simulink model "ss_vec2angles_test"  (R2018b)
settings: Solver=VariableStepAuto  StartTime=0.0  StopTime=10.0  RelTol=1e-3
libraries: vrlib x2, ss_angles_2_vec x1, two_norm x1, ss_vec_2_angles x1
settings Model: Creator=Taylor  LastModifiedBy=Taylor

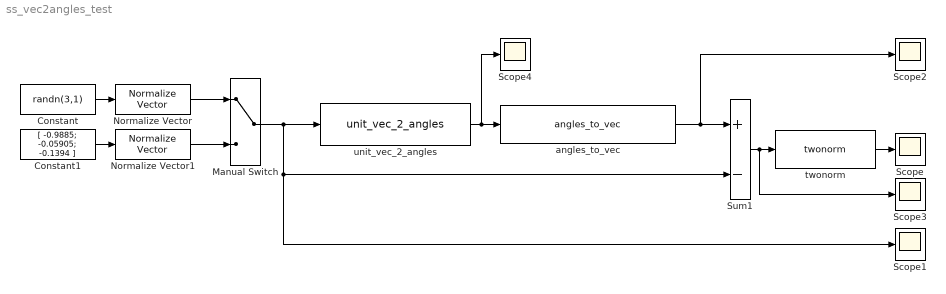
== system ss_vec2angles_test ==
  Constant : Constant  Value=randn(3,1)
  Constant1 : Constant  Value=[ -0.9885; -0.05905; -0.1394 ]
  Manual Switch : ManualSwitch
  Normalize Vector : vrlib/Utilities/Normalize Vector  maxzero=0
      settings: SourceProductName=Simulink 3D Animation  SourceProductBaseCode=VR
  Normalize Vector1 : vrlib/Utilities/Normalize Vector  maxzero=0
      settings: SourceProductName=Simulink 3D Animation  SourceProductBaseCode=VR
  Scope{,1..4} (5 alike) : Scope
  Sum1 : Sum  Inputs=+-
  angles_to_vec : ss_angles_2_vec/angles_to_vec  SystemSampleTime=-1
  twonorm : two_norm/twonorm  SystemSampleTime=-1
  unit_vec_2_angles : ss_vec_2_angles/unit_vec_2_angles  SystemSampleTime=-1
  wires:
  unit_vec_2_angles/1 -> Scope4/1, angles_to_vec/1
  Sum1/1 -> Scope3/1, twonorm/1
  twonorm/1 -> Scope/1
  angles_to_vec/1 -> Scope2/1, Sum1/1
  Manual Switch/1 -> Scope1/1, Sum1/2, unit_vec_2_angles/1
  Normalize Vector/1 -> Manual Switch/1
  Constant1/1 -> Normalize Vector1/1
  Normalize Vector1/1 -> Manual Switch/2
  Constant/1 -> Normalize Vector/1
